simulink model "Battery_model"  (R2021b)
settings: Solver=FixedStepAuto  StartTime=0.0  StopTime=mdl_input.t(end)  FixedStep=1  RelTol=1e-3
values from neighbouring files (symbols this model uses):
  params =     [cell_param.mat]
undefined symbols (not defined in the file or in its folder): mdl_input
libraries: fl_lib x78, nesl_utility x77, simulink x14, ee_lib x14
(part 1 of 2)
settings Model: Creator=pacio  LastModifiedBy=pacio

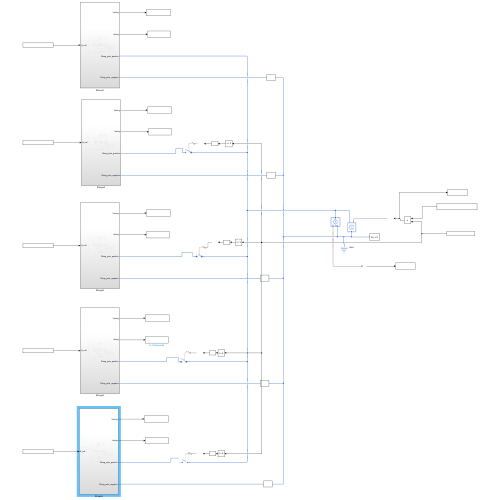
[thumbnail: Simulink's stored preview of the top-level diagram]
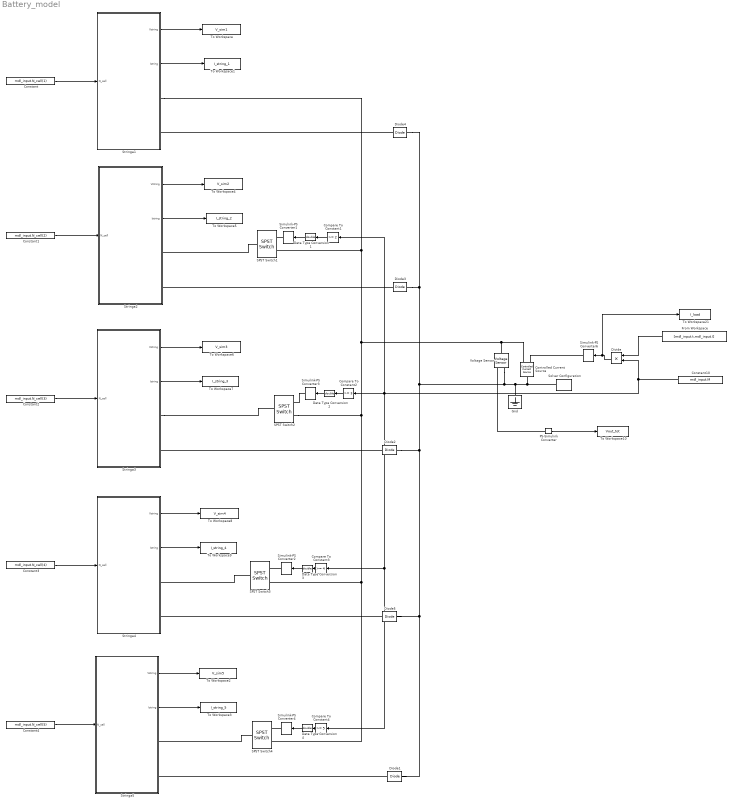
== system Battery_model ==
  Compare To Constant1 : simulink/Logic and Bit Operations/Compare To Constant  relop=>=  const=2  OutDataTypeStr=uint8
  Compare To Constant2 : simulink/Logic and Bit Operations/Compare To Constant  relop=>=  const=3  OutDataTypeStr=uint8
  Compare To Constant3 : simulink/Logic and Bit Operations/Compare To Constant  relop=>=  const=4  OutDataTypeStr=uint8
  Compare To Constant4 : simulink/Logic and Bit Operations/Compare To Constant  relop=>=  const=5  OutDataTypeStr=uint8
  Constant : Constant  Value=mdl_input.N_cell(1)
  Constant1 : Constant  Value=mdl_input.N_cell(2)
  Constant10 : Constant  Value=mdl_input.M
  Constant2 : Constant  Value=mdl_input.N_cell(3)
  Constant3 : Constant  Value=mdl_input.N_cell(4)
  Constant4 : Constant  Value=mdl_input.N_cell(5)
  Controlled Current Source : fl_lib/Electrical/Electrical Sources/Controlled Current Source
  Data Type Conversion{1..4} (4 alike) : DataTypeConversion  OutDataTypeStr=double
  Diode{1..5} (5 alike) : fl_lib/Electrical/Electrical Elements/Diode  Vf=10 mV  Ron=5e-3 Ohm  Goff=1e-5 1/Ohm  i_specify=off  i_priority=High  i=0 A  i_nominal_specify=off  i_nominal_unit=A  i_nominal_value=1  v_specify=off  v_priority=High  v=0 V  v_nominal_specify=off  v_nominal_unit=V  v_nominal_value=1
  Divide : Product  Inputs=**
  From Workspace : FromWorkspace  VariableName=[mdl_input.t,mdl_input.I]
  Gnd : fl_lib/Electrical/Electrical Elements/Electrical Reference
  PS-Simulink Converter : nesl_utility/PS-Simulink Converter  PhysicalDomain=network_engine_domain  SubClassName=ps_output  LeftPortType=input  RightPortType=output  PseudoPeriodic=off  Frequencies=[]  Unit=inherit  AffineConversion=off
      settings: SourceProductBaseCode=PW,SS
  SPST Switch{1..4} (4 alike) : ee_lib/Switches & Breakers/SPST Switch  R_closed=1e-6 Ohm  G_open=1e-6 S  Threshold=0.5 V  Width=0 V  model_dynamics=0  t_on=1e-3 s  t_off=1e-3 s  initial_vT=0 V
      settings: SourceProductBaseCode=PS  InternalSimscapePortConfiguration="{\"Bottom\":[],\"Left\":[{\"id\":\"vT\",\"label\":\"vT\",\"type\":\"input\"},{\"id\":\"p\",\"label\":\"\",\"type\":\"foundation.electrical.electrical\"}],\"Right\":[{\"id\":\"n\",\"label\":\"\",\"type\":\"foundation.electrical.electrical\"}],\"Top\":[]}"
  Simulink-PS Converter{1..4} (4 alike) : nesl_utility/Simulink-PS Converter  PhysicalDomain=network_engine_domain  SubClassName=ps_input  LeftPortType=input  RightPortType=output  PseudoPeriodic=off  Frequencies=[]  NoiseDistribution=none  NoiseParameters=[]  Unit=V  AffineConversion=off  FilteringAndDerivatives=zero  SimscapeFilterOrder=1  InputFilterTimeConstant=0.001  UdotUserProvided=1
  Simulink-PS Converter6 : nesl_utility/Simulink-PS Converter  PhysicalDomain=network_engine_domain  SubClassName=ps_input  LeftPortType=input  RightPortType=output  PseudoPeriodic=off  Frequencies=[]  NoiseDistribution=none  NoiseParameters=[]  Unit=A  AffineConversion=off  FilteringAndDerivatives=zero  SimscapeFilterOrder=1  InputFilterTimeConstant=0.001  UdotUserProvided=1
  Solver Configuration : nesl_utility/Solver Configuration  PhysicalDomain=network_engine_domain  SubClassName=solver  LeftPortType=input  RightPortType=generic  Tones=[]  Harmonics=[]  SimulateNoise=off  Profile=off  UseLocalSampling=off  EnableSwitchedLinearOptims=on  FrequencyDomain=off  UseCCode=off  RelTol=0.001  AbsTol=1e-06  MinStep=1e-09  ToWorkspace=off  RevertToSquareIcSolve=off  NumHomotopyIterations=100  PhasorMode=off  PhasorModeNumHarmonics=1  DoDC=off  ResidualTolerance=1e-09  UseLocalSolver=off  LocalSolverChoice=NE_BACKWARD_EULER_ADVANCER  LocalSolverSampleTime=0.001  DoFixedCost=off  MaxNonlinIter=3  MaxModeIter=2  ComputeImpulses=off  ImpulseIterations=2  LinearAlgebra=Sparse  EquationFormulation=NE_TIME_EF  DelaysMemoryBudget=1024  AutomaticFiltering=on  FilteringTimeConstant=0.001  PartitionStorageMethod=AS_NEEDED  PartitionMemoryBudget=1024  PartitionMethod=FAST
  Stringa1 : Subsystem
  Stringa2 : Subsystem
  Stringa3 : Subsystem
  Stringa4 : Subsystem
  Stringa5 : Subsystem
  To Workspace : ToWorkspace  VariableName=V_sim1  SampleTime=-1
  To Workspace1 : ToWorkspace  VariableName=I_string_1  SampleTime=-1
  To Workspace10 : ToWorkspace  VariableName=Vout_tot  SampleTime=-1
  To Workspace2 : ToWorkspace  VariableName=V_sim5  SampleTime=-1
  To Workspace21 : ToWorkspace  VariableName=I_load  SampleTime=-1
  To Workspace3 : ToWorkspace  VariableName=I_string_5  SampleTime=-1
  To Workspace4 : ToWorkspace  VariableName=V_sim2  SampleTime=-1
  To Workspace5 : ToWorkspace  VariableName=I_string_2  SampleTime=-1
  To Workspace6 : ToWorkspace  VariableName=V_sim3  SampleTime=-1
  To Workspace7 : ToWorkspace  VariableName=I_string_3  SampleTime=-1
  To Workspace8 : ToWorkspace  VariableName=V_sim4  SampleTime=-1
  To Workspace9 : ToWorkspace  VariableName=I_string_4  SampleTime=-1
  Voltage Sensor : fl_lib/Electrical/Electrical Sensors/Voltage Sensor
  wires:
  Stringa1/2(Istring) -> To Workspace1/1
  Stringa1/1(Vstring) -> To Workspace/1
  Constant/1 -> Stringa1/1(N_cell)
  Constant4/1 -> Stringa5/1(N_cell)
  Constant3/1 -> Stringa4/1(N_cell)
  Constant2/1 -> Stringa3/1(N_cell)
  Constant1/1 -> Stringa2/1(N_cell)
  Stringa2/1(Vstring) -> To Workspace4/1
  Stringa2/2(Istring) -> To Workspace5/1
  Stringa3/1(Vstring) -> To Workspace6/1
  Stringa3/2(Istring) -> To Workspace7/1
  Stringa4/1(Vstring) -> To Workspace8/1
  Stringa4/2(Istring) -> To Workspace9/1
  Stringa5/1(Vstring) -> To Workspace2/1
  Stringa5/2(Istring) -> To Workspace3/1
  PS-Simulink Converter/1 -> To Workspace10/1
  From Workspace/1 -> Divide/1
  Divide/1 -> To Workspace21/1, Simulink-PS Converter6/1
  Constant10/1 -> Compare To Constant3/1, Compare To Constant4/1, Compare To Constant1/1, Compare To Constant2/1, Divide/2
  Data Type Conversion2/1 -> Simulink-PS Converter3/1
  Compare To Constant2/1 -> Data Type Conversion2/1
  Data Type Conversion1/1 -> Simulink-PS Converter1/1
  Compare To Constant1/1 -> Data Type Conversion1/1
  Data Type Conversion3/1 -> Simulink-PS Converter2/1
  Compare To Constant3/1 -> Data Type Conversion3/1
  Data Type Conversion4/1 -> Simulink-PS Converter4/1
  Compare To Constant4/1 -> Data Type Conversion4/1
  connections:
  Controlled Current Source/RConn1 -- Simulink-PS Converter6/RConn1
  Diode2/LConn1 -- Diode5/LConn1 -- Diode1/LConn1 -- Diode4/LConn1 -- Diode3/LConn1 -- Solver Configuration/RConn1 -- Controlled Current Source/LConn1 -- Gnd/LConn1 -- Voltage Sensor/RConn2
  Diode1/RConn1 -- Stringa5/RConn2
  Diode5/RConn1 -- Stringa4/RConn2
  Diode2/RConn1 -- Stringa3/RConn2
  Diode3/RConn1 -- Stringa2/RConn2
  Diode4/RConn1 -- Stringa1/RConn2
  PS-Simulink Converter/LConn1 -- Voltage Sensor/RConn1
  SPST Switch1/RConn1 -- Stringa2/RConn1
  Simulink-PS Converter3/RConn1 -- SPST Switch2/LConn1
  Stringa3/RConn1 -- SPST Switch2/RConn1
  Simulink-PS Converter1/RConn1 -- SPST Switch1/LConn1
  Stringa1/RConn1 -- SPST Switch2/LConn2 -- SPST Switch3/LConn2 -- SPST Switch4/LConn2 -- Controlled Current Source/RConn2 -- Voltage Sensor/LConn1 -- SPST Switch1/LConn2
  Simulink-PS Converter2/RConn1 -- SPST Switch3/LConn1
  SPST Switch3/RConn1 -- Stringa4/RConn1
  Simulink-PS Converter4/RConn1 -- SPST Switch4/LConn1
  SPST Switch4/RConn1 -- Stringa5/RConn1

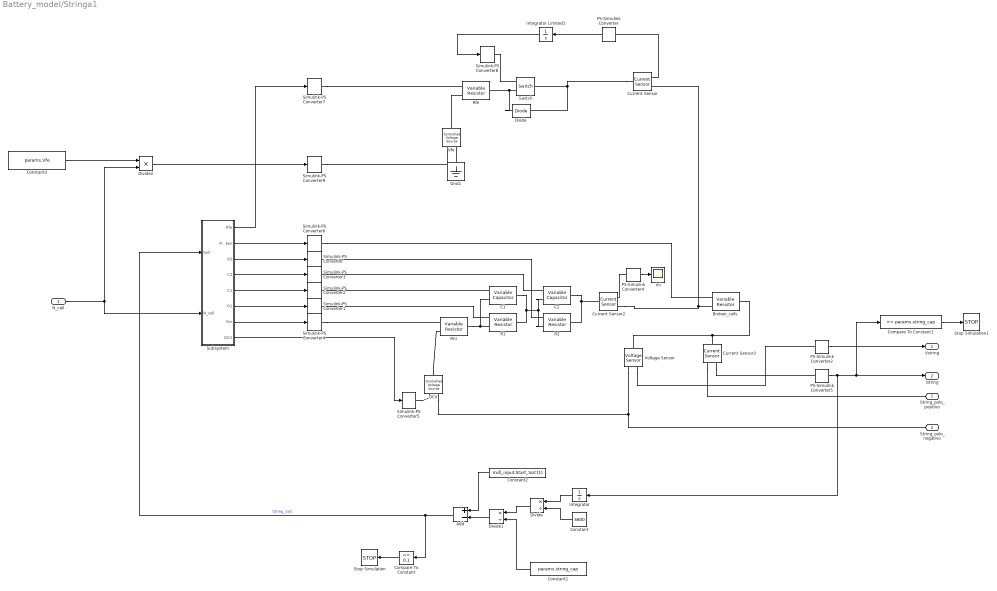
== system Battery_model/Stringa1 ==
  N_cell : Inport
  Add : Sum  Inputs=+-
  Broken_cells : fl_lib/Electrical/Electrical Elements/Variable Resistor  Rmin=0 Ohm  i_specify=off  i_priority=High  i=0 A  i_nominal_specify=off  i_nominal_unit=A  i_nominal_value=1  v_specify=off  v_priority=High  v=0 V  v_nominal_specify=off  v_nominal_unit=V  v_nominal_value=1
  C1 : ee_lib/Passive/Variable Capacitor  prm=2  Cmin=1e-9 F  r=1e-6 Ohm  v0=0 V  q0=0 c
      settings: SourceProductBaseCode=PS  InternalSimscapePortConfiguration="{\"Bottom\":[],\"Left\":[{\"id\":\"C\",\"label\":\"C\",\"type\":\"input\"},{\"id\":\"p\",\"label\":\"+\",\"type\":\"foundation.electrical.electrical\"}],\"Right\":[{\"id\":\"n\",\"label\":\"-\",\"type\":\"foundation.electrical.electrical\"}],\"Top\":[]}"
  C2 : ee_lib/Passive/Variable Capacitor  prm=2  Cmin=1e-9 F  r=1e-6 Ohm  v0=0 V  q0=0 c
      settings: SourceProductBaseCode=PS  InternalSimscapePortConfiguration="{\"Bottom\":[],\"Left\":[{\"id\":\"C\",\"label\":\"C\",\"type\":\"input\"},{\"id\":\"p\",\"label\":\"+\",\"type\":\"foundation.electrical.electrical\"}],\"Right\":[{\"id\":\"n\",\"label\":\"-\",\"type\":\"foundation.electrical.electrical\"}],\"Top\":[]}"
  Compare To Constant : simulink/Logic and Bit Operations/Compare To Constant  relop=<=  const=0.1  OutDataTypeStr=boolean
  Compare To Constant1 : simulink/Logic and Bit Operations/Compare To Constant  relop=>=  const=params.string_cap  OutDataTypeStr=boolean
  Constant : Constant  Value=3600
  Constant1 : Constant  Value=params.string_cap
  Constant2 : Constant  Value=mdl_input.Start_SoC(1)
  Constant3 : Constant  Value=params.Vfe
  Current Sensor : fl_lib/Electrical/Electrical Sensors/Current Sensor
  Current Sensor2 : fl_lib/Electrical/Electrical Sensors/Current Sensor
  Current Sensor3 : fl_lib/Electrical/Electrical Sensors/Current Sensor
  Diode : fl_lib/Electrical/Electrical Elements/Diode  Vf=1 mV  Ron=1e-5 Ohm  Goff=1e-5 1/Ohm  i_specify=off  i_priority=High  i=0 A  i_nominal_specify=off  i_nominal_unit=A  i_nominal_value=1  v_specify=off  v_priority=High  v=0 V  v_nominal_specify=off  v_nominal_unit=V  v_nominal_value=1
  Divide : Product  Inputs=*/
  Divide1 : Product  Inputs=*/
  Divide2 : Product  Inputs=**
  Gnd1 : fl_lib/Electrical/Electrical Elements/Electrical Reference
  Ini : Scope
  Integrator : Integrator
  Integrator Limited1 : Integrator  UpperSaturationLimit=0.9  LowerSaturationLimit=0.1
  OCV : fl_lib/Electrical/Electrical Sources/Controlled Voltage Source
  PS-Simulink Converter{,2,4..5} (4 alike) : nesl_utility/PS-Simulink Converter  PhysicalDomain=network_engine_domain  SubClassName=ps_output  LeftPortType=input  RightPortType=output  PseudoPeriodic=off  Frequencies=[]  Unit=1  AffineConversion=off
  R1 : fl_lib/Electrical/Electrical Elements/Variable Resistor  Rmin=0 Ohm  i_specify=off  i_priority=High  i=0 A  i_nominal_specify=off  i_nominal_unit=A  i_nominal_value=1  v_specify=off  v_priority=High  v=0 V  v_nominal_specify=off  v_nominal_unit=V  v_nominal_value=1
  R2 : fl_lib/Electrical/Electrical Elements/Variable Resistor  Rmin=0 Ohm  i_specify=off  i_priority=High  i=0 A  i_nominal_specify=off  i_nominal_unit=A  i_nominal_value=1  v_specify=off  v_priority=High  v=0 V  v_nominal_specify=off  v_nominal_unit=V  v_nominal_value=1
  Rfe : fl_lib/Electrical/Electrical Elements/Variable Resistor  Rmin=0 Ohm  i_specify=off  i_priority=High  i=0 A  i_nominal_specify=off  i_nominal_unit=A  i_nominal_value=1  v_specify=off  v_priority=High  v=0 V  v_nominal_specify=off  v_nominal_unit=V  v_nominal_value=1
  Rni : fl_lib/Electrical/Electrical Elements/Variable Resistor  Rmin=0 Ohm  i_specify=off  i_priority=High  i=0 A  i_nominal_specify=off  i_nominal_unit=A  i_nominal_value=1  v_specify=off  v_priority=High  v=0 V  v_nominal_specify=off  v_nominal_unit=V  v_nominal_value=1
  Simulink-PS Converter{,1..4,6..9} (9 alike) : nesl_utility/Simulink-PS Converter  PhysicalDomain=network_engine_domain  SubClassName=ps_input  LeftPortType=input  RightPortType=output  PseudoPeriodic=off  Frequencies=[]  NoiseDistribution=none  NoiseParameters=[]  Unit=1  AffineConversion=off  FilteringAndDerivatives=zero  SimscapeFilterOrder=1  InputFilterTimeConstant=0.001  UdotUserProvided=1
  Simulink-PS Converter5 : nesl_utility/Simulink-PS Converter  PhysicalDomain=network_engine_domain  SubClassName=ps_input  LeftPortType=input  RightPortType=output  PseudoPeriodic=off  Frequencies=[]  NoiseDistribution=none  NoiseParameters=[]  Unit=V  AffineConversion=off  FilteringAndDerivatives=zero  SimscapeFilterOrder=1  InputFilterTimeConstant=0.001  UdotUserProvided=1
  Stop Simulation : Stop
  Stop Simulation1 : Stop
  Subsystem : Subsystem
  Switch : fl_lib/Electrical/Electrical Elements/Switch  R_closed=1e-6 Ohm  G_open=1e-6 1/Ohm  Threshold=0.1  i_specify=off  i_priority=High  i=0 A  i_nominal_specify=off  i_nominal_unit=A  i_nominal_value=1  v_specify=off  v_priority=High  v=0 V  v_nominal_specify=off  v_nominal_unit=V  v_nominal_value=1
  Vfe : fl_lib/Electrical/Electrical Sources/Controlled Voltage Source
  Voltage Sensor : fl_lib/Electrical/Electrical Sensors/Voltage Sensor
  String_polo_positivo : PMIOPort  Side=Right
  String_polo_negativo : PMIOPort  Port=2  Side=Right
  Vstring : Outport
  Istring : Outport  Port=2
  wires:
  Subsystem/1(Rfe) -> Simulink-PS Converter7/1
  Subsystem/8(OCV) -> Simulink-PS Converter5/1
  PS-Simulink Converter/1 -> Integrator Limited1/1
  Subsystem/7(Rni) -> Simulink-PS Converter4/1
  Subsystem/6(R1) -> Simulink-PS Converter1/1
  PS-Simulink Converter2/1 -> Vstring/1
  PS-Simulink Converter4/1 -> Ini/1
  Integrator Limited1/1 -> Simulink-PS Converter8/1
  PS-Simulink Converter5/1 -> Compare To Constant1/1, Istring/1, Integrator/1
  Subsystem/5(C1) -> Simulink-PS Converter2/1
  Subsystem/3(R2) -> Simulink-PS Converter/1
  Add/1 -> Compare To Constant/1, Subsystem/1(SoC)  "String_SoC"
  Subsystem/4(C2) -> Simulink-PS Converter3/1
  N_cell/1 -> Divide2/2, Subsystem/2(N_cell)
  Integrator/1 -> Divide/1
  Constant/1 -> Divide/2
  Divide/1 -> Divide1/1
  Constant1/1 -> Divide1/2
  Divide1/1 -> Add/2
  Constant2/1 -> Add/1
  Subsystem/2(Rbroken) -> Simulink-PS Converter6/1
  Divide2/1 -> Simulink-PS Converter9/1
  Constant3/1 -> Divide2/1
  Compare To Constant/1 -> Stop Simulation/1
  Compare To Constant1/1 -> Stop Simulation1/1
  connections:
  Current Sensor2/RConn2 -- Broken_cells/LConn2 -- Current Sensor/RConn2
  Current Sensor2/LConn1 -- R2/RConn1 -- C2/RConn1
  OCV/RConn2 -- Voltage Sensor/RConn2 -- String_polo_negativo/RConn1
  Simulink-PS Converter3/RConn1 -- C2/LConn1
  OCV/LConn1 -- Rni/LConn2
  Simulink-PS Converter7/RConn1 -- Rfe/LConn1
  Simulink-PS Converter2/RConn1 -- C1/LConn1
  Vfe/LConn1 -- Rfe/LConn2
  Current Sensor/LConn1 -- Diode/RConn1 -- Switch/LConn1
  C2/LConn2 -- R2/LConn2 -- R1/RConn1 -- C1/RConn1
  Simulink-PS Converter/RConn1 -- R2/LConn1
  Simulink-PS Converter8/RConn1 -- Switch/RConn1
  Rni/RConn1 -- R1/LConn2 -- C1/LConn2
  Voltage Sensor/RConn1 -- PS-Simulink Converter2/LConn1
  Diode/LConn1 -- Rfe/RConn1 -- Switch/RConn2
  PS-Simulink Converter4/LConn1 -- Current Sensor2/RConn1
  Simulink-PS Converter4/RConn1 -- Rni/LConn1
  Simulink-PS Converter1/RConn1 -- R1/LConn1
  Current Sensor3/RConn2 -- String_polo_positivo/RConn1
  Gnd1/LConn1 -- Vfe/RConn2
  Simulink-PS Converter5/RConn1 -- OCV/RConn1
  Current Sensor/RConn1 -- PS-Simulink Converter/LConn1
  Current Sensor3/RConn1 -- PS-Simulink Converter5/LConn1
  Broken_cells/RConn1 -- Voltage Sensor/LConn1 -- Current Sensor3/LConn1
  Simulink-PS Converter6/RConn1 -- Broken_cells/LConn1
  Simulink-PS Converter9/RConn1 -- Vfe/RConn1

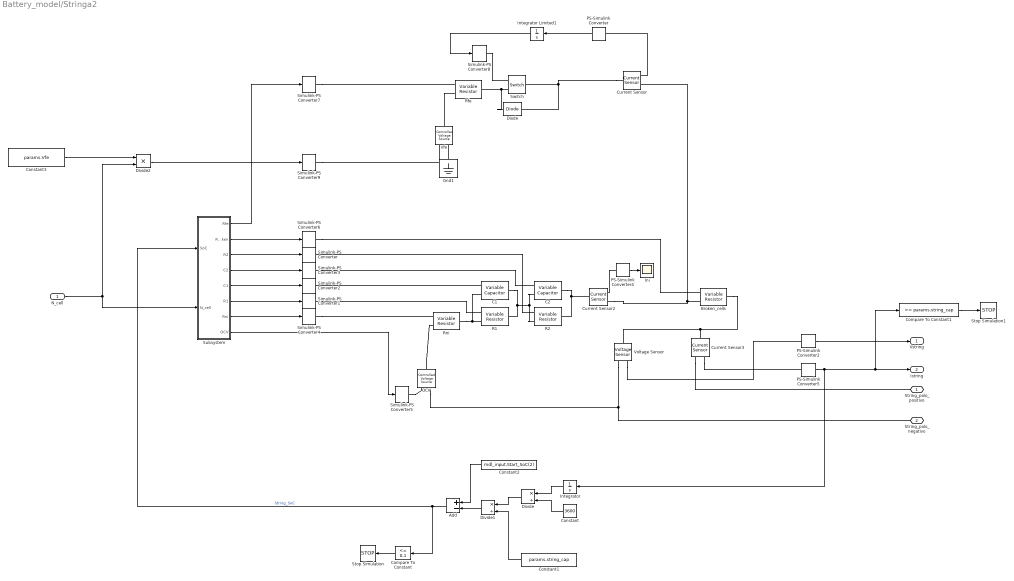
== system Battery_model/Stringa2 ==
  N_cell : Inport
  Add : Sum  Inputs=+-
  Broken_cells : fl_lib/Electrical/Electrical Elements/Variable Resistor  Rmin=0 Ohm  i_specify=off  i_priority=High  i=0 A  i_nominal_specify=off  i_nominal_unit=A  i_nominal_value=1  v_specify=off  v_priority=High  v=0 V  v_nominal_specify=off  v_nominal_unit=V  v_nominal_value=1
  C1 : ee_lib/Passive/Variable Capacitor  prm=2  Cmin=1e-9 F  r=1e-6 Ohm  v0=0 V  q0=0 c
      settings: SourceProductBaseCode=PS  InternalSimscapePortConfiguration="{\"Bottom\":[],\"Left\":[{\"id\":\"C\",\"label\":\"C\",\"type\":\"input\"},{\"id\":\"p\",\"label\":\"+\",\"type\":\"foundation.electrical.electrical\"}],\"Right\":[{\"id\":\"n\",\"label\":\"-\",\"type\":\"foundation.electrical.electrical\"}],\"Top\":[]}"
  C2 : ee_lib/Passive/Variable Capacitor  prm=2  Cmin=1e-9 F  r=1e-6 Ohm  v0=0 V  q0=0 c
      settings: SourceProductBaseCode=PS  InternalSimscapePortConfiguration="{\"Bottom\":[],\"Left\":[{\"id\":\"C\",\"label\":\"C\",\"type\":\"input\"},{\"id\":\"p\",\"label\":\"+\",\"type\":\"foundation.electrical.electrical\"}],\"Right\":[{\"id\":\"n\",\"label\":\"-\",\"type\":\"foundation.electrical.electrical\"}],\"Top\":[]}"
  Compare To Constant : simulink/Logic and Bit Operations/Compare To Constant  relop=<=  const=0.1  OutDataTypeStr=boolean
  Compare To Constant1 : simulink/Logic and Bit Operations/Compare To Constant  relop=>=  const=params.string_cap  OutDataTypeStr=boolean
  Constant : Constant  Value=3600
  Constant1 : Constant  Value=params.string_cap
  Constant2 : Constant  Value=mdl_input.Start_SoC(2)
  Constant3 : Constant  Value=params.Vfe
  Current Sensor : fl_lib/Electrical/Electrical Sensors/Current Sensor
  Current Sensor2 : fl_lib/Electrical/Electrical Sensors/Current Sensor
  Current Sensor3 : fl_lib/Electrical/Electrical Sensors/Current Sensor
  Diode : fl_lib/Electrical/Electrical Elements/Diode  Vf=1 mV  Ron=1e-5 Ohm  Goff=1e-5 1/Ohm  i_specify=off  i_priority=High  i=0 A  i_nominal_specify=off  i_nominal_unit=A  i_nominal_value=1  v_specify=off  v_priority=High  v=0 V  v_nominal_specify=off  v_nominal_unit=V  v_nominal_value=1
  Divide : Product  Inputs=*/
  Divide1 : Product  Inputs=*/
  Divide2 : Product  Inputs=**
  Gnd1 : fl_lib/Electrical/Electrical Elements/Electrical Reference
  Ini : Scope
  Integrator : Integrator
  Integrator Limited1 : Integrator  UpperSaturationLimit=0.9  LowerSaturationLimit=0.1
  OCV : fl_lib/Electrical/Electrical Sources/Controlled Voltage Source
  PS-Simulink Converter{,2,4..5} (4 alike) : nesl_utility/PS-Simulink Converter  PhysicalDomain=network_engine_domain  SubClassName=ps_output  LeftPortType=input  RightPortType=output  PseudoPeriodic=off  Frequencies=[]  Unit=1  AffineConversion=off
  R1 : fl_lib/Electrical/Electrical Elements/Variable Resistor  Rmin=0 Ohm  i_specify=off  i_priority=High  i=0 A  i_nominal_specify=off  i_nominal_unit=A  i_nominal_value=1  v_specify=off  v_priority=High  v=0 V  v_nominal_specify=off  v_nominal_unit=V  v_nominal_value=1
  R2 : fl_lib/Electrical/Electrical Elements/Variable Resistor  Rmin=0 Ohm  i_specify=off  i_priority=High  i=0 A  i_nominal_specify=off  i_nominal_unit=A  i_nominal_value=1  v_specify=off  v_priority=High  v=0 V  v_nominal_specify=off  v_nominal_unit=V  v_nominal_value=1
  Rfe : fl_lib/Electrical/Electrical Elements/Variable Resistor  Rmin=0 Ohm  i_specify=off  i_priority=High  i=0 A  i_nominal_specify=off  i_nominal_unit=A  i_nominal_value=1  v_specify=off  v_priority=High  v=0 V  v_nominal_specify=off  v_nominal_unit=V  v_nominal_value=1
  Rni : fl_lib/Electrical/Electrical Elements/Variable Resistor  Rmin=0 Ohm  i_specify=off  i_priority=High  i=0 A  i_nominal_specify=off  i_nominal_unit=A  i_nominal_value=1  v_specify=off  v_priority=High  v=0 V  v_nominal_specify=off  v_nominal_unit=V  v_nominal_value=1
  Simulink-PS Converter{,1..4,6..9} (9 alike) : nesl_utility/Simulink-PS Converter  PhysicalDomain=network_engine_domain  SubClassName=ps_input  LeftPortType=input  RightPortType=output  PseudoPeriodic=off  Frequencies=[]  NoiseDistribution=none  NoiseParameters=[]  Unit=1  AffineConversion=off  FilteringAndDerivatives=zero  SimscapeFilterOrder=1  InputFilterTimeConstant=0.001  UdotUserProvided=1
  Simulink-PS Converter5 : nesl_utility/Simulink-PS Converter  PhysicalDomain=network_engine_domain  SubClassName=ps_input  LeftPortType=input  RightPortType=output  PseudoPeriodic=off  Frequencies=[]  NoiseDistribution=none  NoiseParameters=[]  Unit=V  AffineConversion=off  FilteringAndDerivatives=zero  SimscapeFilterOrder=1  InputFilterTimeConstant=0.001  UdotUserProvided=1
  Stop Simulation : Stop
  Stop Simulation1 : Stop
  Subsystem : Subsystem
  Switch : fl_lib/Electrical/Electrical Elements/Switch  R_closed=1e-6 Ohm  G_open=1e-6 1/Ohm  Threshold=0.1  i_specify=off  i_priority=High  i=0 A  i_nominal_specify=off  i_nominal_unit=A  i_nominal_value=1  v_specify=off  v_priority=High  v=0 V  v_nominal_specify=off  v_nominal_unit=V  v_nominal_value=1
  Vfe : fl_lib/Electrical/Electrical Sources/Controlled Voltage Source
  Voltage Sensor : fl_lib/Electrical/Electrical Sensors/Voltage Sensor
  String_polo_positivo : PMIOPort  Side=Right
  String_polo_negativo : PMIOPort  Port=2  Side=Right
  Vstring : Outport
  Istring : Outport  Port=2
  wires:
  Subsystem/1(Rfe) -> Simulink-PS Converter7/1
  Subsystem/8(OCV) -> Simulink-PS Converter5/1
  PS-Simulink Converter/1 -> Integrator Limited1/1
  Subsystem/7(Rni) -> Simulink-PS Converter4/1
  Subsystem/6(R1) -> Simulink-PS Converter1/1
  PS-Simulink Converter2/1 -> Vstring/1
  PS-Simulink Converter4/1 -> Ini/1
  Integrator Limited1/1 -> Simulink-PS Converter8/1
  Subsystem/5(C1) -> Simulink-PS Converter2/1
  Subsystem/3(R2) -> Simulink-PS Converter/1
  Subsystem/4(C2) -> Simulink-PS Converter3/1
  N_cell/1 -> Divide2/2, Subsystem/2(N_cell)
  Integrator/1 -> Divide/1
  Constant/1 -> Divide/2
  Divide/1 -> Divide1/1
  Constant1/1 -> Divide1/2
  Divide1/1 -> Add/2
  Constant2/1 -> Add/1
  Subsystem/2(Rbroken) -> Simulink-PS Converter6/1
  Divide2/1 -> Simulink-PS Converter9/1
  Constant3/1 -> Divide2/1
  Compare To Constant/1 -> Stop Simulation/1
  Add/1 -> Compare To Constant/1, Subsystem/1(SoC)  "String_SoC"
  PS-Simulink Converter5/1 -> Compare To Constant1/1, Istring/1, Integrator/1
  Compare To Constant1/1 -> Stop Simulation1/1
  connections:
  Current Sensor2/RConn2 -- Broken_cells/LConn2 -- Current Sensor/RConn2
  Current Sensor2/LConn1 -- R2/RConn1 -- C2/RConn1
  OCV/RConn2 -- Voltage Sensor/RConn2 -- String_polo_negativo/RConn1
  Simulink-PS Converter3/RConn1 -- C2/LConn1
  OCV/LConn1 -- Rni/LConn2
  Simulink-PS Converter7/RConn1 -- Rfe/LConn1
  Simulink-PS Converter2/RConn1 -- C1/LConn1
  Vfe/LConn1 -- Rfe/LConn2
  Current Sensor/LConn1 -- Switch/LConn1 -- Diode/RConn1
  C2/LConn2 -- R2/LConn2 -- R1/RConn1 -- C1/RConn1
  Simulink-PS Converter/RConn1 -- R2/LConn1
  Simulink-PS Converter8/RConn1 -- Switch/RConn1
  Rni/RConn1 -- R1/LConn2 -- C1/LConn2
  Voltage Sensor/RConn1 -- PS-Simulink Converter2/LConn1
  Diode/LConn1 -- Rfe/RConn1 -- Switch/RConn2
  PS-Simulink Converter4/LConn1 -- Current Sensor2/RConn1
  Simulink-PS Converter4/RConn1 -- Rni/LConn1
  Simulink-PS Converter1/RConn1 -- R1/LConn1
  Current Sensor3/RConn2 -- String_polo_positivo/RConn1
  Gnd1/LConn1 -- Vfe/RConn2
  Simulink-PS Converter5/RConn1 -- OCV/RConn1
  Current Sensor/RConn1 -- PS-Simulink Converter/LConn1
  Current Sensor3/RConn1 -- PS-Simulink Converter5/LConn1
  Broken_cells/RConn1 -- Voltage Sensor/LConn1 -- Current Sensor3/LConn1
  Simulink-PS Converter6/RConn1 -- Broken_cells/LConn1
  Simulink-PS Converter9/RConn1 -- Vfe/RConn1

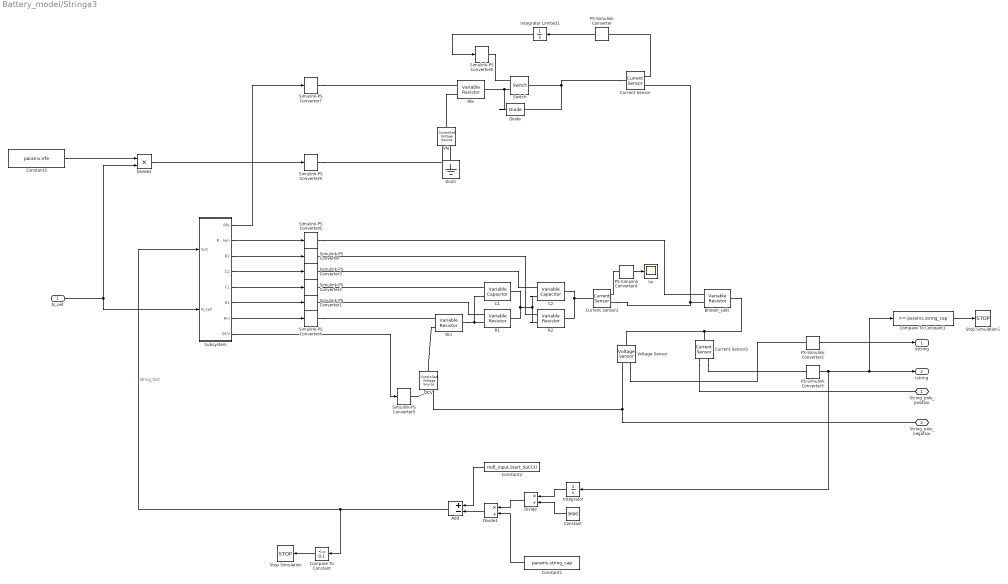
== system Battery_model/Stringa3 ==
  N_cell : Inport
  Add : Sum  Inputs=+-
  Broken_cells : fl_lib/Electrical/Electrical Elements/Variable Resistor  Rmin=0 Ohm  i_specify=off  i_priority=High  i=0 A  i_nominal_specify=off  i_nominal_unit=A  i_nominal_value=1  v_specify=off  v_priority=High  v=0 V  v_nominal_specify=off  v_nominal_unit=V  v_nominal_value=1
  C1 : ee_lib/Passive/Variable Capacitor  prm=2  Cmin=1e-9 F  r=1e-6 Ohm  v0=0 V  q0=0 c
      settings: SourceProductBaseCode=PS  InternalSimscapePortConfiguration="{\"Bottom\":[],\"Left\":[{\"id\":\"C\",\"label\":\"C\",\"type\":\"input\"},{\"id\":\"p\",\"label\":\"+\",\"type\":\"foundation.electrical.electrical\"}],\"Right\":[{\"id\":\"n\",\"label\":\"-\",\"type\":\"foundation.electrical.electrical\"}],\"Top\":[]}"
  C2 : ee_lib/Passive/Variable Capacitor  prm=2  Cmin=1e-9 F  r=1e-6 Ohm  v0=0 V  q0=0 c
      settings: SourceProductBaseCode=PS  InternalSimscapePortConfiguration="{\"Bottom\":[],\"Left\":[{\"id\":\"C\",\"label\":\"C\",\"type\":\"input\"},{\"id\":\"p\",\"label\":\"+\",\"type\":\"foundation.electrical.electrical\"}],\"Right\":[{\"id\":\"n\",\"label\":\"-\",\"type\":\"foundation.electrical.electrical\"}],\"Top\":[]}"
  Compare To Constant : simulink/Logic and Bit Operations/Compare To Constant  relop=<=  const=0.1  OutDataTypeStr=boolean
  Compare To Constant1 : simulink/Logic and Bit Operations/Compare To Constant  relop=>=  const=params.string_cap  OutDataTypeStr=boolean
  Constant : Constant  Value=3600
  Constant1 : Constant  Value=params.string_cap
  Constant2 : Constant  Value=mdl_input.Start_SoC(3)
  Constant3 : Constant  Value=params.Vfe
  Current Sensor : fl_lib/Electrical/Electrical Sensors/Current Sensor
  Current Sensor2 : fl_lib/Electrical/Electrical Sensors/Current Sensor
  Current Sensor3 : fl_lib/Electrical/Electrical Sensors/Current Sensor
  Diode : fl_lib/Electrical/Electrical Elements/Diode  Vf=1 mV  Ron=1e-5 Ohm  Goff=1e-5 1/Ohm  i_specify=off  i_priority=High  i=0 A  i_nominal_specify=off  i_nominal_unit=A  i_nominal_value=1  v_specify=off  v_priority=High  v=0 V  v_nominal_specify=off  v_nominal_unit=V  v_nominal_value=1
  Divide : Product  Inputs=*/
  Divide1 : Product  Inputs=*/
  Divide2 : Product  Inputs=**
  Gnd1 : fl_lib/Electrical/Electrical Elements/Electrical Reference
  Ini : Scope
  Integrator : Integrator
  Integrator Limited1 : Integrator  UpperSaturationLimit=0.9  LowerSaturationLimit=0.1
  OCV : fl_lib/Electrical/Electrical Sources/Controlled Voltage Source
  PS-Simulink Converter{,2,4..5} (4 alike) : nesl_utility/PS-Simulink Converter  PhysicalDomain=network_engine_domain  SubClassName=ps_output  LeftPortType=input  RightPortType=output  PseudoPeriodic=off  Frequencies=[]  Unit=1  AffineConversion=off
  R1 : fl_lib/Electrical/Electrical Elements/Variable Resistor  Rmin=0 Ohm  i_specify=off  i_priority=High  i=0 A  i_nominal_specify=off  i_nominal_unit=A  i_nominal_value=1  v_specify=off  v_priority=High  v=0 V  v_nominal_specify=off  v_nominal_unit=V  v_nominal_value=1
  R2 : fl_lib/Electrical/Electrical Elements/Variable Resistor  Rmin=0 Ohm  i_specify=off  i_priority=High  i=0 A  i_nominal_specify=off  i_nominal_unit=A  i_nominal_value=1  v_specify=off  v_priority=High  v=0 V  v_nominal_specify=off  v_nominal_unit=V  v_nominal_value=1
  Rfe : fl_lib/Electrical/Electrical Elements/Variable Resistor  Rmin=0 Ohm  i_specify=off  i_priority=High  i=0 A  i_nominal_specify=off  i_nominal_unit=A  i_nominal_value=1  v_specify=off  v_priority=High  v=0 V  v_nominal_specify=off  v_nominal_unit=V  v_nominal_value=1
  Rni : fl_lib/Electrical/Electrical Elements/Variable Resistor  Rmin=0 Ohm  i_specify=off  i_priority=High  i=0 A  i_nominal_specify=off  i_nominal_unit=A  i_nominal_value=1  v_specify=off  v_priority=High  v=0 V  v_nominal_specify=off  v_nominal_unit=V  v_nominal_value=1
  Simulink-PS Converter{,1..4,6..9} (9 alike) : nesl_utility/Simulink-PS Converter  PhysicalDomain=network_engine_domain  SubClassName=ps_input  LeftPortType=input  RightPortType=output  PseudoPeriodic=off  Frequencies=[]  NoiseDistribution=none  NoiseParameters=[]  Unit=1  AffineConversion=off  FilteringAndDerivatives=zero  SimscapeFilterOrder=1  InputFilterTimeConstant=0.001  UdotUserProvided=1
  Simulink-PS Converter5 : nesl_utility/Simulink-PS Converter  PhysicalDomain=network_engine_domain  SubClassName=ps_input  LeftPortType=input  RightPortType=output  PseudoPeriodic=off  Frequencies=[]  NoiseDistribution=none  NoiseParameters=[]  Unit=V  AffineConversion=off  FilteringAndDerivatives=zero  SimscapeFilterOrder=1  InputFilterTimeConstant=0.001  UdotUserProvided=1
  Stop Simulation : Stop
  Stop Simulation1 : Stop
  Subsystem : Subsystem
  Switch : fl_lib/Electrical/Electrical Elements/Switch  R_closed=1e-6 Ohm  G_open=1e-6 1/Ohm  Threshold=0.1  i_specify=off  i_priority=High  i=0 A  i_nominal_specify=off  i_nominal_unit=A  i_nominal_value=1  v_specify=off  v_priority=High  v=0 V  v_nominal_specify=off  v_nominal_unit=V  v_nominal_value=1
  Vfe : fl_lib/Electrical/Electrical Sources/Controlled Voltage Source
  Voltage Sensor : fl_lib/Electrical/Electrical Sensors/Voltage Sensor
  String_polo_positivo : PMIOPort  Side=Right
  String_polo_negativo : PMIOPort  Port=2  Side=Right
  Vstring : Outport
  Istring : Outport  Port=2
  wires:
  Subsystem/1(Rfe) -> Simulink-PS Converter7/1
  Subsystem/8(OCV) -> Simulink-PS Converter5/1
  PS-Simulink Converter/1 -> Integrator Limited1/1
  Subsystem/7(Rni) -> Simulink-PS Converter4/1
  Subsystem/6(R1) -> Simulink-PS Converter1/1
  PS-Simulink Converter2/1 -> Vstring/1
  PS-Simulink Converter4/1 -> Ini/1
  Integrator Limited1/1 -> Simulink-PS Converter8/1
  Subsystem/5(C1) -> Simulink-PS Converter2/1
  Subsystem/3(R2) -> Simulink-PS Converter/1
  Subsystem/4(C2) -> Simulink-PS Converter3/1
  N_cell/1 -> Divide2/2, Subsystem/2(N_cell)
  Integrator/1 -> Divide/1
  Constant/1 -> Divide/2
  Divide/1 -> Divide1/1
  Constant1/1 -> Divide1/2
  Divide1/1 -> Add/2
  Constant2/1 -> Add/1
  Subsystem/2(Rbroken) -> Simulink-PS Converter6/1
  Divide2/1 -> Simulink-PS Converter9/1
  Constant3/1 -> Divide2/1
  Compare To Constant/1 -> Stop Simulation/1
  Add/1 -> Compare To Constant/1, Subsystem/1(SoC)  "String_SoC"
  PS-Simulink Converter5/1 -> Compare To Constant1/1, Istring/1, Integrator/1
  Compare To Constant1/1 -> Stop Simulation1/1
  connections:
  Current Sensor2/RConn2 -- Broken_cells/LConn2 -- Current Sensor/RConn2
  Current Sensor2/LConn1 -- R2/RConn1 -- C2/RConn1
  OCV/RConn2 -- Voltage Sensor/RConn2 -- String_polo_negativo/RConn1
  Simulink-PS Converter3/RConn1 -- C2/LConn1
  OCV/LConn1 -- Rni/LConn2
  Simulink-PS Converter7/RConn1 -- Rfe/LConn1
  Simulink-PS Converter2/RConn1 -- C1/LConn1
  Vfe/LConn1 -- Rfe/LConn2
  Current Sensor/LConn1 -- Switch/LConn1 -- Diode/RConn1
  C2/LConn2 -- R2/LConn2 -- R1/RConn1 -- C1/RConn1
  Simulink-PS Converter/RConn1 -- R2/LConn1
  Simulink-PS Converter8/RConn1 -- Switch/RConn1
  Rni/RConn1 -- R1/LConn2 -- C1/LConn2
  Voltage Sensor/RConn1 -- PS-Simulink Converter2/LConn1
  Diode/LConn1 -- Rfe/RConn1 -- Switch/RConn2
  PS-Simulink Converter4/LConn1 -- Current Sensor2/RConn1
  Simulink-PS Converter4/RConn1 -- Rni/LConn1
  Simulink-PS Converter1/RConn1 -- R1/LConn1
  Current Sensor3/RConn2 -- String_polo_positivo/RConn1
  Gnd1/LConn1 -- Vfe/RConn2
  Simulink-PS Converter5/RConn1 -- OCV/RConn1
  Current Sensor/RConn1 -- PS-Simulink Converter/LConn1
  Current Sensor3/RConn1 -- PS-Simulink Converter5/LConn1
  Broken_cells/RConn1 -- Voltage Sensor/LConn1 -- Current Sensor3/LConn1
  Simulink-PS Converter6/RConn1 -- Broken_cells/LConn1
  Simulink-PS Converter9/RConn1 -- Vfe/RConn1

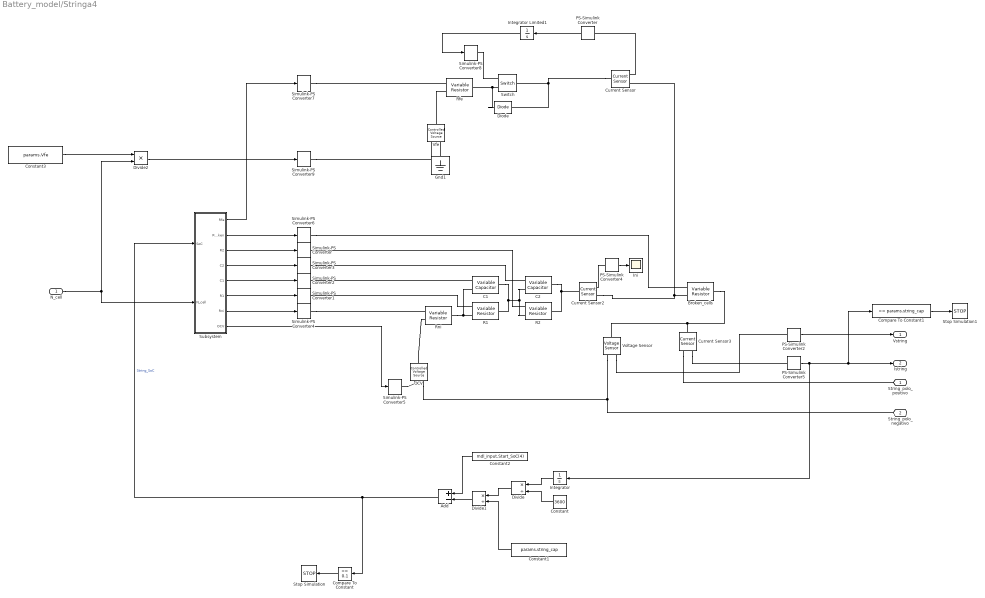
== system Battery_model/Stringa4 ==
  N_cell : Inport
  Add : Sum  Inputs=+-
  Broken_cells : fl_lib/Electrical/Electrical Elements/Variable Resistor  Rmin=0 Ohm  i_specify=off  i_priority=High  i=0 A  i_nominal_specify=off  i_nominal_unit=A  i_nominal_value=1  v_specify=off  v_priority=High  v=0 V  v_nominal_specify=off  v_nominal_unit=V  v_nominal_value=1
  C1 : ee_lib/Passive/Variable Capacitor  prm=2  Cmin=1e-9 F  r=1e-6 Ohm  v0=0 V  q0=0 c
      settings: SourceProductBaseCode=PS  InternalSimscapePortConfiguration="{\"Bottom\":[],\"Left\":[{\"id\":\"C\",\"label\":\"C\",\"type\":\"input\"},{\"id\":\"p\",\"label\":\"+\",\"type\":\"foundation.electrical.electrical\"}],\"Right\":[{\"id\":\"n\",\"label\":\"-\",\"type\":\"foundation.electrical.electrical\"}],\"Top\":[]}"
  C2 : ee_lib/Passive/Variable Capacitor  prm=2  Cmin=1e-9 F  r=1e-6 Ohm  v0=0 V  q0=0 c
      settings: SourceProductBaseCode=PS  InternalSimscapePortConfiguration="{\"Bottom\":[],\"Left\":[{\"id\":\"C\",\"label\":\"C\",\"type\":\"input\"},{\"id\":\"p\",\"label\":\"+\",\"type\":\"foundation.electrical.electrical\"}],\"Right\":[{\"id\":\"n\",\"label\":\"-\",\"type\":\"foundation.electrical.electrical\"}],\"Top\":[]}"
  Compare To Constant : simulink/Logic and Bit Operations/Compare To Constant  relop=<=  const=0.1  OutDataTypeStr=boolean
  Compare To Constant1 : simulink/Logic and Bit Operations/Compare To Constant  relop=>=  const=params.string_cap  OutDataTypeStr=boolean
  Constant : Constant  Value=3600
  Constant1 : Constant  Value=params.string_cap
  Constant2 : Constant  Value=mdl_input.Start_SoC(4)
  Constant3 : Constant  Value=params.Vfe
  Current Sensor : fl_lib/Electrical/Electrical Sensors/Current Sensor
  Current Sensor2 : fl_lib/Electrical/Electrical Sensors/Current Sensor
  Current Sensor3 : fl_lib/Electrical/Electrical Sensors/Current Sensor
  Diode : fl_lib/Electrical/Electrical Elements/Diode  Vf=1 mV  Ron=1e-5 Ohm  Goff=1e-5 1/Ohm  i_specify=off  i_priority=High  i=0 A  i_nominal_specify=off  i_nominal_unit=A  i_nominal_value=1  v_specify=off  v_priority=High  v=0 V  v_nominal_specify=off  v_nominal_unit=V  v_nominal_value=1
  Divide : Product  Inputs=*/
  Divide1 : Product  Inputs=*/
  Divide2 : Product  Inputs=**
  Gnd1 : fl_lib/Electrical/Electrical Elements/Electrical Reference
  Ini : Scope
  Integrator : Integrator
  Integrator Limited1 : Integrator  UpperSaturationLimit=0.9  LowerSaturationLimit=0.1
  OCV : fl_lib/Electrical/Electrical Sources/Controlled Voltage Source
  PS-Simulink Converter{,2,4..5} (4 alike) : nesl_utility/PS-Simulink Converter  PhysicalDomain=network_engine_domain  SubClassName=ps_output  LeftPortType=input  RightPortType=output  PseudoPeriodic=off  Frequencies=[]  Unit=1  AffineConversion=off
  R1 : fl_lib/Electrical/Electrical Elements/Variable Resistor  Rmin=0 Ohm  i_specify=off  i_priority=High  i=0 A  i_nominal_specify=off  i_nominal_unit=A  i_nominal_value=1  v_specify=off  v_priority=High  v=0 V  v_nominal_specify=off  v_nominal_unit=V  v_nominal_value=1
  R2 : fl_lib/Electrical/Electrical Elements/Variable Resistor  Rmin=0 Ohm  i_specify=off  i_priority=High  i=0 A  i_nominal_specify=off  i_nominal_unit=A  i_nominal_value=1  v_specify=off  v_priority=High  v=0 V  v_nominal_specify=off  v_nominal_unit=V  v_nominal_value=1
  Rfe : fl_lib/Electrical/Electrical Elements/Variable Resistor  Rmin=0 Ohm  i_specify=off  i_priority=High  i=0 A  i_nominal_specify=off  i_nominal_unit=A  i_nominal_value=1  v_specify=off  v_priority=High  v=0 V  v_nominal_specify=off  v_nominal_unit=V  v_nominal_value=1
  Rni : fl_lib/Electrical/Electrical Elements/Variable Resistor  Rmin=0 Ohm  i_specify=off  i_priority=High  i=0 A  i_nominal_specify=off  i_nominal_unit=A  i_nominal_value=1  v_specify=off  v_priority=High  v=0 V  v_nominal_specify=off  v_nominal_unit=V  v_nominal_value=1
  Simulink-PS Converter{,1..4,6..9} (9 alike) : nesl_utility/Simulink-PS Converter  PhysicalDomain=network_engine_domain  SubClassName=ps_input  LeftPortType=input  RightPortType=output  PseudoPeriodic=off  Frequencies=[]  NoiseDistribution=none  NoiseParameters=[]  Unit=1  AffineConversion=off  FilteringAndDerivatives=zero  SimscapeFilterOrder=1  InputFilterTimeConstant=0.001  UdotUserProvided=1
  Simulink-PS Converter5 : nesl_utility/Simulink-PS Converter  PhysicalDomain=network_engine_domain  SubClassName=ps_input  LeftPortType=input  RightPortType=output  PseudoPeriodic=off  Frequencies=[]  NoiseDistribution=none  NoiseParameters=[]  Unit=V  AffineConversion=off  FilteringAndDerivatives=zero  SimscapeFilterOrder=1  InputFilterTimeConstant=0.001  UdotUserProvided=1
  Stop Simulation : Stop
  Stop Simulation1 : Stop
  Subsystem : Subsystem
  Switch : fl_lib/Electrical/Electrical Elements/Switch  R_closed=1e-6 Ohm  G_open=1e-6 1/Ohm  Threshold=0.1  i_specify=off  i_priority=High  i=0 A  i_nominal_specify=off  i_nominal_unit=A  i_nominal_value=1  v_specify=off  v_priority=High  v=0 V  v_nominal_specify=off  v_nominal_unit=V  v_nominal_value=1
  Vfe : fl_lib/Electrical/Electrical Sources/Controlled Voltage Source
  Voltage Sensor : fl_lib/Electrical/Electrical Sensors/Voltage Sensor
  String_polo_positivo : PMIOPort  Side=Right
  String_polo_negativo : PMIOPort  Port=2  Side=Right
  Vstring : Outport
  Istring : Outport  Port=2
  wires:
  Subsystem/1(Rfe) -> Simulink-PS Converter7/1
  Subsystem/8(OCV) -> Simulink-PS Converter5/1
  PS-Simulink Converter/1 -> Integrator Limited1/1
  Subsystem/7(Rni) -> Simulink-PS Converter4/1
  Subsystem/6(R1) -> Simulink-PS Converter1/1
  PS-Simulink Converter2/1 -> Vstring/1
  PS-Simulink Converter4/1 -> Ini/1
  Integrator Limited1/1 -> Simulink-PS Converter8/1
  Subsystem/5(C1) -> Simulink-PS Converter2/1
  Subsystem/3(R2) -> Simulink-PS Converter/1
  Subsystem/4(C2) -> Simulink-PS Converter3/1
  N_cell/1 -> Divide2/2, Subsystem/2(N_cell)
  Integrator/1 -> Divide/1
  Constant/1 -> Divide/2
  Divide/1 -> Divide1/1
  Constant1/1 -> Divide1/2
  Divide1/1 -> Add/2
  Constant2/1 -> Add/1
  Subsystem/2(Rbroken) -> Simulink-PS Converter6/1
  Divide2/1 -> Simulink-PS Converter9/1
  Constant3/1 -> Divide2/1
  Compare To Constant/1 -> Stop Simulation/1
  Add/1 -> Compare To Constant/1, Subsystem/1(SoC)  "String_SoC"
  PS-Simulink Converter5/1 -> Compare To Constant1/1, Istring/1, Integrator/1
  Compare To Constant1/1 -> Stop Simulation1/1
  connections:
  Current Sensor2/RConn2 -- Broken_cells/LConn2 -- Current Sensor/RConn2
  Current Sensor2/LConn1 -- R2/RConn1 -- C2/RConn1
  OCV/RConn2 -- Voltage Sensor/RConn2 -- String_polo_negativo/RConn1
  Simulink-PS Converter3/RConn1 -- C2/LConn1
  OCV/LConn1 -- Rni/LConn2
  Simulink-PS Converter7/RConn1 -- Rfe/LConn1
  Simulink-PS Converter2/RConn1 -- C1/LConn1
  Vfe/LConn1 -- Rfe/LConn2
  Current Sensor/LConn1 -- Switch/LConn1 -- Diode/RConn1
  C2/LConn2 -- R2/LConn2 -- R1/RConn1 -- C1/RConn1
  Simulink-PS Converter/RConn1 -- R2/LConn1
  Simulink-PS Converter8/RConn1 -- Switch/RConn1
  Rni/RConn1 -- R1/LConn2 -- C1/LConn2
  Voltage Sensor/RConn1 -- PS-Simulink Converter2/LConn1
  Diode/LConn1 -- Rfe/RConn1 -- Switch/RConn2
  PS-Simulink Converter4/LConn1 -- Current Sensor2/RConn1
  Simulink-PS Converter4/RConn1 -- Rni/LConn1
  Simulink-PS Converter1/RConn1 -- R1/LConn1
  Current Sensor3/RConn2 -- String_polo_positivo/RConn1
  Gnd1/LConn1 -- Vfe/RConn2
  Simulink-PS Converter5/RConn1 -- OCV/RConn1
  Current Sensor/RConn1 -- PS-Simulink Converter/LConn1
  Current Sensor3/RConn1 -- PS-Simulink Converter5/LConn1
  Broken_cells/RConn1 -- Voltage Sensor/LConn1 -- Current Sensor3/LConn1
  Simulink-PS Converter6/RConn1 -- Broken_cells/LConn1
  Simulink-PS Converter9/RConn1 -- Vfe/RConn1

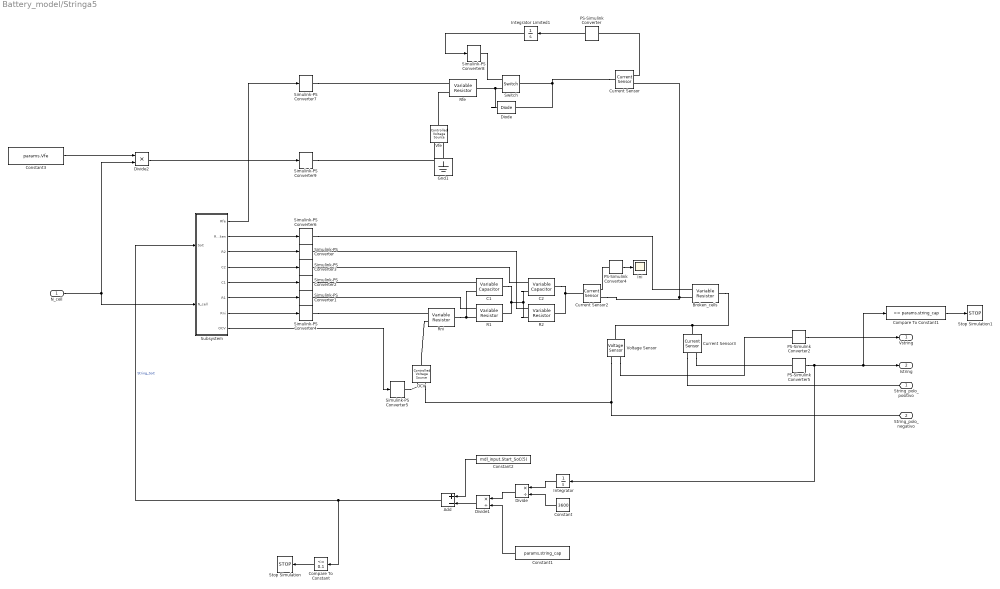
== system Battery_model/Stringa5 ==
  N_cell : Inport
  Add : Sum  Inputs=+-
  Broken_cells : fl_lib/Electrical/Electrical Elements/Variable Resistor  Rmin=0 Ohm  i_specify=off  i_priority=High  i=0 A  i_nominal_specify=off  i_nominal_unit=A  i_nominal_value=1  v_specify=off  v_priority=High  v=0 V  v_nominal_specify=off  v_nominal_unit=V  v_nominal_value=1
  C1 : ee_lib/Passive/Variable Capacitor  prm=2  Cmin=1e-9 F  r=1e-6 Ohm  v0=0 V  q0=0 c
      settings: SourceProductBaseCode=PS  InternalSimscapePortConfiguration="{\"Bottom\":[],\"Left\":[{\"id\":\"C\",\"label\":\"C\",\"type\":\"input\"},{\"id\":\"p\",\"label\":\"+\",\"type\":\"foundation.electrical.electrical\"}],\"Right\":[{\"id\":\"n\",\"label\":\"-\",\"type\":\"foundation.electrical.electrical\"}],\"Top\":[]}"
  C2 : ee_lib/Passive/Variable Capacitor  prm=2  Cmin=1e-9 F  r=1e-6 Ohm  v0=0 V  q0=0 c
      settings: SourceProductBaseCode=PS  InternalSimscapePortConfiguration="{\"Bottom\":[],\"Left\":[{\"id\":\"C\",\"label\":\"C\",\"type\":\"input\"},{\"id\":\"p\",\"label\":\"+\",\"type\":\"foundation.electrical.electrical\"}],\"Right\":[{\"id\":\"n\",\"label\":\"-\",\"type\":\"foundation.electrical.electrical\"}],\"Top\":[]}"
  Compare To Constant : simulink/Logic and Bit Operations/Compare To Constant  relop=<=  const=0.1  OutDataTypeStr=boolean
  Compare To Constant1 : simulink/Logic and Bit Operations/Compare To Constant  relop=>=  const=params.string_cap  OutDataTypeStr=boolean
  Constant : Constant  Value=3600
  Constant1 : Constant  Value=params.string_cap
  Constant2 : Constant  Value=mdl_input.Start_SoC(5)
  Constant3 : Constant  Value=params.Vfe
  Current Sensor : fl_lib/Electrical/Electrical Sensors/Current Sensor
  Current Sensor2 : fl_lib/Electrical/Electrical Sensors/Current Sensor
  Current Sensor3 : fl_lib/Electrical/Electrical Sensors/Current Sensor
  Diode : fl_lib/Electrical/Electrical Elements/Diode  Vf=1 mV  Ron=1e-5 Ohm  Goff=1e-5 1/Ohm  i_specify=off  i_priority=High  i=0 A  i_nominal_specify=off  i_nominal_unit=A  i_nominal_value=1  v_specify=off  v_priority=High  v=0 V  v_nominal_specify=off  v_nominal_unit=V  v_nominal_value=1
  Divide : Product  Inputs=*/
  Divide1 : Product  Inputs=*/
  Divide2 : Product  Inputs=**
  Gnd1 : fl_lib/Electrical/Electrical Elements/Electrical Reference
  Ini : Scope
  Integrator : Integrator
  Integrator Limited1 : Integrator  UpperSaturationLimit=0.9  LowerSaturationLimit=0.1
  OCV : fl_lib/Electrical/Electrical Sources/Controlled Voltage Source
  PS-Simulink Converter{,2,4..5} (4 alike) : nesl_utility/PS-Simulink Converter  PhysicalDomain=network_engine_domain  SubClassName=ps_output  LeftPortType=input  RightPortType=output  PseudoPeriodic=off  Frequencies=[]  Unit=1  AffineConversion=off
  R1 : fl_lib/Electrical/Electrical Elements/Variable Resistor  Rmin=0 Ohm  i_specify=off  i_priority=High  i=0 A  i_nominal_specify=off  i_nominal_unit=A  i_nominal_value=1  v_specify=off  v_priority=High  v=0 V  v_nominal_specify=off  v_nominal_unit=V  v_nominal_value=1
  R2 : fl_lib/Electrical/Electrical Elements/Variable Resistor  Rmin=0 Ohm  i_specify=off  i_priority=High  i=0 A  i_nominal_specify=off  i_nominal_unit=A  i_nominal_value=1  v_specify=off  v_priority=High  v=0 V  v_nominal_specify=off  v_nominal_unit=V  v_nominal_value=1
  Rfe : fl_lib/Electrical/Electrical Elements/Variable Resistor  Rmin=0 Ohm  i_specify=off  i_priority=High  i=0 A  i_nominal_specify=off  i_nominal_unit=A  i_nominal_value=1  v_specify=off  v_priority=High  v=0 V  v_nominal_specify=off  v_nominal_unit=V  v_nominal_value=1
  Rni : fl_lib/Electrical/Electrical Elements/Variable Resistor  Rmin=0 Ohm  i_specify=off  i_priority=High  i=0 A  i_nominal_specify=off  i_nominal_unit=A  i_nominal_value=1  v_specify=off  v_priority=High  v=0 V  v_nominal_specify=off  v_nominal_unit=V  v_nominal_value=1
  Simulink-PS Converter{,1..4,6..9} (9 alike) : nesl_utility/Simulink-PS Converter  PhysicalDomain=network_engine_domain  SubClassName=ps_input  LeftPortType=input  RightPortType=output  PseudoPeriodic=off  Frequencies=[]  NoiseDistribution=none  NoiseParameters=[]  Unit=1  AffineConversion=off  FilteringAndDerivatives=zero  SimscapeFilterOrder=1  InputFilterTimeConstant=0.001  UdotUserProvided=1
  Simulink-PS Converter5 : nesl_utility/Simulink-PS Converter  PhysicalDomain=network_engine_domain  SubClassName=ps_input  LeftPortType=input  RightPortType=output  PseudoPeriodic=off  Frequencies=[]  NoiseDistribution=none  NoiseParameters=[]  Unit=V  AffineConversion=off  FilteringAndDerivatives=zero  SimscapeFilterOrder=1  InputFilterTimeConstant=0.001  UdotUserProvided=1
  Stop Simulation : Stop
  Stop Simulation1 : Stop
  Subsystem : Subsystem
  Switch : fl_lib/Electrical/Electrical Elements/Switch  R_closed=1e-6 Ohm  G_open=1e-6 1/Ohm  Threshold=0.1  i_specify=off  i_priority=High  i=0 A  i_nominal_specify=off  i_nominal_unit=A  i_nominal_value=1  v_specify=off  v_priority=High  v=0 V  v_nominal_specify=off  v_nominal_unit=V  v_nominal_value=1
  Vfe : fl_lib/Electrical/Electrical Sources/Controlled Voltage Source
  Voltage Sensor : fl_lib/Electrical/Electrical Sensors/Voltage Sensor
  String_polo_positivo : PMIOPort  Side=Right
  String_polo_negativo : PMIOPort  Port=2  Side=Right
  Vstring : Outport
  Istring : Outport  Port=2
  wires:
  Subsystem/1(Rfe) -> Simulink-PS Converter7/1
  Subsystem/8(OCV) -> Simulink-PS Converter5/1
  PS-Simulink Converter/1 -> Integrator Limited1/1
  Subsystem/7(Rni) -> Simulink-PS Converter4/1
  Subsystem/6(R1) -> Simulink-PS Converter1/1
  PS-Simulink Converter2/1 -> Vstring/1
  PS-Simulink Converter4/1 -> Ini/1
  Integrator Limited1/1 -> Simulink-PS Converter8/1
  Subsystem/5(C1) -> Simulink-PS Converter2/1
  Subsystem/3(R2) -> Simulink-PS Converter/1
  Subsystem/4(C2) -> Simulink-PS Converter3/1
  N_cell/1 -> Divide2/2, Subsystem/2(N_cell)
  Integrator/1 -> Divide/1
  Constant/1 -> Divide/2
  Divide/1 -> Divide1/1
  Constant1/1 -> Divide1/2
  Divide1/1 -> Add/2
  Constant2/1 -> Add/1
  Subsystem/2(Rbroken) -> Simulink-PS Converter6/1
  Divide2/1 -> Simulink-PS Converter9/1
  Constant3/1 -> Divide2/1
  Compare To Constant/1 -> Stop Simulation/1
  Add/1 -> Compare To Constant/1, Subsystem/1(SoC)  "String_SoC"
  PS-Simulink Converter5/1 -> Compare To Constant1/1, Istring/1, Integrator/1
  Compare To Constant1/1 -> Stop Simulation1/1
  connections:
  Current Sensor2/RConn2 -- Broken_cells/LConn2 -- Current Sensor/RConn2
  Current Sensor2/LConn1 -- R2/RConn1 -- C2/RConn1
  OCV/RConn2 -- Voltage Sensor/RConn2 -- String_polo_negativo/RConn1
  Simulink-PS Converter3/RConn1 -- C2/LConn1
  OCV/LConn1 -- Rni/LConn2
  Simulink-PS Converter7/RConn1 -- Rfe/LConn1
  Simulink-PS Converter2/RConn1 -- C1/LConn1
  Vfe/LConn1 -- Rfe/LConn2
  Current Sensor/LConn1 -- Switch/LConn1 -- Diode/RConn1
  C2/LConn2 -- R2/LConn2 -- R1/RConn1 -- C1/RConn1
  Simulink-PS Converter/RConn1 -- R2/LConn1
  Simulink-PS Converter8/RConn1 -- Switch/RConn1
  Rni/RConn1 -- R1/LConn2 -- C1/LConn2
  Voltage Sensor/RConn1 -- PS-Simulink Converter2/LConn1
  Diode/LConn1 -- Rfe/RConn1 -- Switch/RConn2
  PS-Simulink Converter4/LConn1 -- Current Sensor2/RConn1
  Simulink-PS Converter4/RConn1 -- Rni/LConn1
  Simulink-PS Converter1/RConn1 -- R1/LConn1
  Current Sensor3/RConn2 -- String_polo_positivo/RConn1
  Gnd1/LConn1 -- Vfe/RConn2
  Simulink-PS Converter5/RConn1 -- OCV/RConn1
  Current Sensor/RConn1 -- PS-Simulink Converter/LConn1
  Current Sensor3/RConn1 -- PS-Simulink Converter5/LConn1
  Broken_cells/RConn1 -- Voltage Sensor/LConn1 -- Current Sensor3/LConn1
  Simulink-PS Converter6/RConn1 -- Broken_cells/LConn1
  Simulink-PS Converter9/RConn1 -- Vfe/RConn1

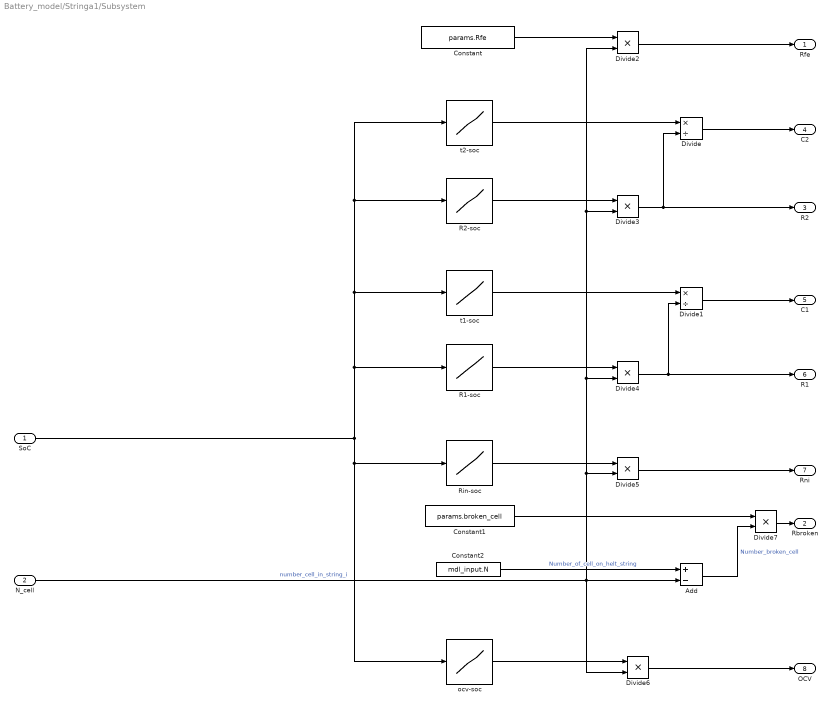
== system Battery_model/Stringa1/Subsystem ==
  SoC : Inport
  N_cell : Inport  Port=2
  Add : Sum  Inputs=+-
  Constant : Constant  Value=params.Rfe
  Constant1 : Constant  Value=params.broken_cell
  Constant2 : Constant  Value=mdl_input.N
  Divide : Product  Inputs=*/
  Divide1 : Product  Inputs=*/
  Divide{2..7} (6 alike) : Product  Inputs=**
  R1-soc : Lookup_n-D  NumberOfTableDimensions=1  BreakpointsForDimension1=params.SoC  Table=params.R1  InternalRulePriority=Speed  RndMeth=Simplest  InputSameDT=on
  R2-soc : Lookup_n-D  NumberOfTableDimensions=1  BreakpointsForDimension1=params.SoC  Table=params.R2  InternalRulePriority=Speed  RndMeth=Simplest  InputSameDT=on
  Rin-soc : Lookup_n-D  NumberOfTableDimensions=1  BreakpointsForDimension1=params.SoC  Table=params.Rni  InternalRulePriority=Speed  RndMeth=Simplest  InputSameDT=on
  ocv-soc : Lookup_n-D  NumberOfTableDimensions=1  BreakpointsForDimension1=params.SoC  Table=params.OCV  ExtrapMethod=Clip  UseLastTableValue=on  InternalRulePriority=Speed  RndMeth=Simplest  InputSameDT=on
  t1-soc : Lookup_n-D  NumberOfTableDimensions=1  BreakpointsForDimension1=params.SoC  Table=params.t1  InternalRulePriority=Speed  RndMeth=Simplest  InputSameDT=on
  t2-soc : Lookup_n-D  NumberOfTableDimensions=1  BreakpointsForDimension1=params.SoC  Table=params.t2  InternalRulePriority=Speed  RndMeth=Simplest  InputSameDT=on
  Rfe : Outport
  Rbroken : Outport  Port=2
  R2 : Outport  Port=3
  C2 : Outport  Port=4
  C1 : Outport  Port=5
  R1 : Outport  Port=6
  Rni : Outport  Port=7
  OCV : Outport  Port=8
  wires:
  SoC/1 -> ocv-soc/1, Rin-soc/1, t1-soc/1, R2-soc/1, t2-soc/1, R1-soc/1
  t1-soc/1 -> Divide1/1
  Divide1/1 -> C1/1
  t2-soc/1 -> Divide/1
  Divide/1 -> C2/1
  Constant/1 -> Divide2/1
  Divide2/1 -> Rfe/1
  R2-soc/1 -> Divide3/1
  Divide3/1 -> Divide/2, R2/1
  Divide4/1 -> Divide1/2, R1/1
  R1-soc/1 -> Divide4/1
  ocv-soc/1 -> Divide6/1
  Divide6/1 -> OCV/1
  Rin-soc/1 -> Divide5/1
  N_cell/1 -> Divide6/2, Add/2, Divide5/2, Divide4/2, Divide3/2, Divide2/2  "number_cell_in_string_i"
  Constant2/1 -> Add/1  "Number_of_cell_on_helt_string"
  Constant1/1 -> Divide7/1
  Add/1 -> Divide7/2  "Number_broken_cell"
  Divide7/1 -> Rbroken/1
  Divide5/1 -> Rni/1
